simulink model "open_loop_simulation"  (R2020b)
settings: Solver=ode45  StartTime=0.0  StopTime=10  FixedStep=0.01  RelTol=1e-3  EnableMultiTasking=on
values from neighbouring files (symbols this model uses):
  Theta1_0 = pi    (= 3.14159265359)    [simulation.m]
  Theta2_0 = -pi/2    (= -1.57079632679)    [simulation.m]
  Thetad1_0 = 0    [simulation.m]
  Thetad2_0 = 0    [simulation.m]
settings Model: Creator=rbabuska  LastModifiedBy=fabia
settings DataIOCC: LimitDataPoints=on  SaveFormat=Array  ReturnWorkspaceOutputs=off  SignalLoggingName=sigsOut
settings OptimizationCC: BooleanDataType=off  ExpressionDepthLimit=2147483647  InitFltsAndDblsToZero=on  LifeSpan=inf
settings DebuggingCC: SaveWithParameterizedLinksMsg=none  SignalResolutionControl=TryResolveAllWithWarning  MultiTaskDSMMsg=warning  MultiTaskCondExecSysMsg=none  AllowSymbolicDim=off  StateNameClashWarn=warning  SFUnexpectedBacktrackingDiag=warning  SFNoUnconditionalDefaultTransitionDiag=warning  SFExecutionAtInitializationDiag=none  ArithmeticOperatorsInVariantConditions=warning
settings HardwareCC: ProdBitPerPointer=32  ProdBitPerSizeT=32  ProdBitPerPtrDiffT=32  ProdLargestAtomicFloat=None  ProdIntDivRoundTo=Undefined  ProdEndianess=Unspecified  ProdWordSize=32  ProdHWDeviceType=32-bit Generic  TargetUnknown=on
settings ModelReferenceCC: PropagateSignalLabelsOutOfModel=off
settings SFSimCC: SimUseLocalCustomCode=off  CustomCodeUndefinedFunction=UseInterfaceOnly
settings RTWCC: RTWUseLocalCustomCode=off
settings CodeAppCC: StateflowObjectComments=on
settings GRTTargetCC: TargetFcnLib=ansi_tfl_tmw.mat  TargetLangStandard=C89/C90 (ANSI)  CombineOutputUpdateFcns=off  GRTInterface=on
settings ConfigComp: CovMetricSettings=dw  CovSaveCumulativeToWorkspaceVar=on  CovSaveSingleToWorkspaceVar=on  CovExternalEMLEnable=off

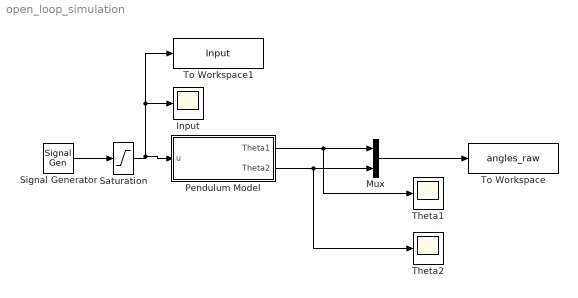
== system open_loop_simulation ==
  Input : Scope
  Mux : Mux  Inputs=2
  Pendulum Model : Subsystem
  Saturation : Saturate  UpperLimit=1  LowerLimit=-1
  Signal Generator : SignalGenerator  Amplitude=0.5  Frequency=5
  Theta1 : Scope
  Theta2 : Scope
  To Workspace : ToWorkspace  VariableName=angles_raw  SaveFormat=Timeseries  SampleTime=-1
  To Workspace1 : ToWorkspace  VariableName=Input  SaveFormat=Timeseries  SampleTime=-1
  wires:
  Saturation/1 -> To Workspace1/1, Input/1, Pendulum Model/1(u)
  Signal Generator/1 -> Saturation/1
  Pendulum Model/1(Theta1) -> Mux/1, Theta1/1
  Pendulum Model/2(Theta2) -> Mux/2, Theta2/1
  Mux/1 -> To Workspace/1

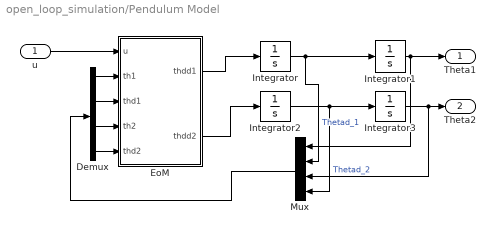
== system open_loop_simulation/Pendulum Model ==
  u : Inport
  Demux : Demux
  EoM : MATLAB Function  TreatAsAtomicUnit=on
  Integrator : Integrator  InitialCondition=Thetad1_0  ContinuousStateAttributes='Theta1'
  Integrator1 : Integrator  InitialCondition=Theta1_0  ContinuousStateAttributes='Theta1'
  Integrator2 : Integrator  InitialCondition=Thetad2_0  ContinuousStateAttributes='Theta1'
  Integrator3 : Integrator  InitialCondition=Theta2_0  ContinuousStateAttributes='Theta1'
  Mux : Mux
  Theta1 : Outport
  Theta2 : Outport  Port=2
  wires:
  Integrator1/1 -> Mux/1, Theta1/1
  Integrator/1 -> Mux/2, Integrator1/1  "Thetad_1"
  EoM/2(thdd2) -> Integrator2/1
  Integrator2/1 -> Mux/4, Integrator3/1  "Thetad_2"
  Integrator3/1 -> Mux/3, Theta2/1
  u/1 -> EoM/1(u)
  EoM/1(thdd1) -> Integrator/1
  Demux/1 -> EoM/2(th1)
  Demux/2 -> EoM/3(thd1)
  Demux/3 -> EoM/4(th2)
  Demux/4 -> EoM/5(thd2)
  Mux/1 -> Demux/1

== matlab function open_loop_simulation/Pendulum Model/EoM ==
  data: u input; thdd1 output; th1 input; thd1 input; th2 input; thd2 input; model_par parameter; thdd2 output
function [thdd1, thdd2] = fcn(u, th1, thd1, th2, thd2, model_par)
thdd1 = 0;
thdd2 = -(model_par.b*thd2 + model_par.c2*model_par.g*model_par.m2*sin(th2))/(model_par.m2*model_par.c2^2 + model_par.J2);
